simulink model "model"  (R2023b)
settings: Solver=VariableStepAuto  StartTime=0.0  StopTime=10.0  RelTol=1e-3
undefined symbols (not defined in the file): DiscIntNeverNeededParam, Newton, Raphson
libraries: simulink x43, slpidlib x11
(part 1 of 2)
settings Model: Creator=OSCAR4  LastModifiedBy=OSCAR4

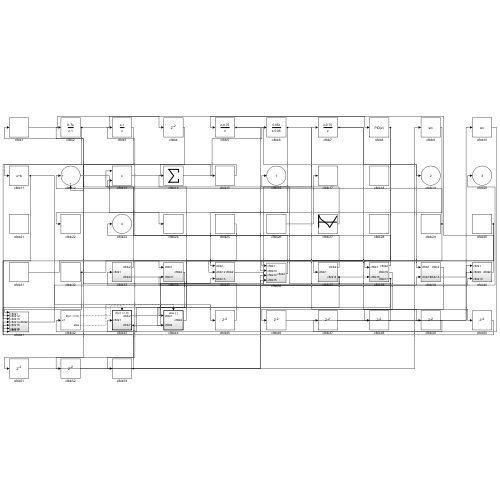
[thumbnail: Simulink's stored preview of the top-level diagram]
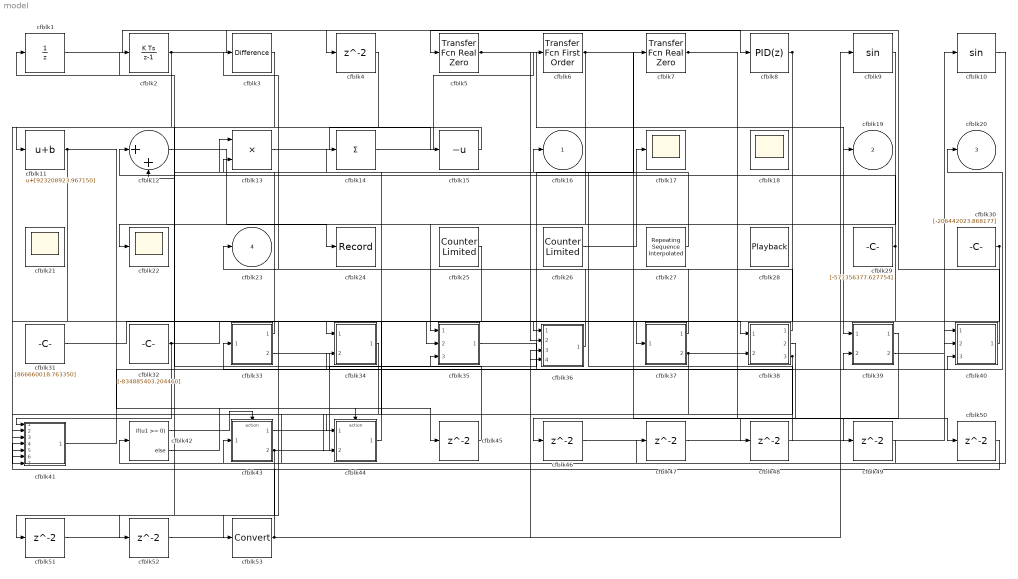
== system model ==
  cfblk1 : UnitDelay  HasFrameUpgradeWarning=on
  cfblk10 : Trigonometry
  cfblk11 : Bias  Bias=[923208923.967150]  SaturateOnIntegerOverflow=off
  cfblk12 : Sum  Inputs=|++
  cfblk13 : Product
  cfblk14 : Sum  Inputs=+
  cfblk15 : UnaryMinus
  cfblk{17..18,21..22} (4 alike) : Scope
      cfblk18 settings: Floating=on
      cfblk21 settings: Floating=on
  cfblk2 : DiscreteIntegrator  ICPrevOutput=DiscIntNeverNeededParam  ICPrevScaledInput=DiscIntNeverNeededParam
  cfblk24 : Record  FileSettingsInternal="{\"entries\":[{\"content\":{\"excelSettings\":{\"content\":{},\"type\":\"Streamout.ExcelSettings\"}},\"type\":\"Streamout.FileSettingStorage\",\"uuid\":\"\"}],\"packageUris\":[\"http:\\/\\/schema.mathworks.com\\/mf0\\/streamout_blocks\\/R2020a\"],\"version\":\"1.0\"}"  SignalsInternal="{\"entries\":[{\"content\":{\"signals\":[{\"content\":{\"blockPath\":[],\"dimensions\":[1],\"domain\":\"\",\"lineColor\":\"#ff6929\",\"plots\":[1],\"port\":1,\"sid\":[\"\"],\"signalID\":3599,\"signalName\":\"cfblk12\"},\"type\":\"RecordBlkView.Signal\",\"uuid\":\"\"}]},\"type\":\"RecordBlkView.InputSignals\",\"uuid\":\"\"}],\"packageUris\":[\"http:\\/\\/schema.mathworks.com\\/mf0\\/streamout_blocks\\/R2020a\"],\"version\":\"1.0\"}"  VisualizationBindings="{\"sparklinesplugin\":{\"info\":[{\"bindingParametersList\":[],\"subplotID\":1}]}}"
  cfblk25 : simulink/Sources/Counter Limited  uplimit=[906.000000]  tsamp=-1
  cfblk26 : simulink/Sources/Counter Limited  uplimit=[721.000000]  tsamp=-1
  cfblk27 : simulink/Sources/Repeating Sequence Interpolated  OutValues=[733850769.124770, 317296340.211416, -269417737.220056, -565735887.153496, 618114081.511135]  TimeValues=[0 0.1 0.5 0.6 1].'  LookUpMeth=Interpolation-Use End Values  tsamp=0.01  OutMin=[]  OutMax=[]  OutDataTypeStr=double  OutputDataTypeScalingMode=double  OutDataType=fixdt(0,8)  OutScaling=2^-10
  cfblk28 : Playback  NumPorts=0  PartName=b20fab14-a049-489c-adbd-99bd70615e82
  cfblk29 : Constant  Value=[-571356377.627754]  SampleTime=1
  cfblk3 : simulink/Discrete/Difference  ICPrevInput=0.0  OutMin=[]  OutMax=[]  OutDataTypeStr=Inherit: Inherit via back propagation  OutDataType=fixdt(1, 16)  OutScaling=2^-10  DoSatur=off
  cfblk30 : Constant  Value=[-206442023.868177]  SampleTime=1
  cfblk31 : Constant  Value=[866660018.763350]  SampleTime=1
  cfblk32 : Constant  Value=[-834885403.204460]  SampleTime=1
  cfblk33 : Subsystem
  cfblk34 : Subsystem
  cfblk35 : Subsystem
  cfblk36 : Subsystem
  cfblk37 : Subsystem
  cfblk38 : Subsystem
  cfblk39 : Subsystem
  cfblk{4,45..52} (9 alike) : Delay  SampleTime=1
  cfblk40 : Subsystem
  cfblk41 : Subsystem
  cfblk42 : If  IfExpression=u1 >= 0  SampleTime=1
  cfblk43 : Subsystem  TreatAsAtomicUnit=on
  cfblk44 : Subsystem  TreatAsAtomicUnit=on
  cfblk5 : simulink/Discrete/Transfer Fcn Real Zero  ZeroZ=0.75  ICPrevInput=0.0  DoSatur=off
  cfblk53 : DataTypeConversion  SaturateOnIntegerOverflow=off  RndMeth=Floor
  cfblk6 : simulink/Discrete/Transfer Fcn First Order  PoleZ=0.95  ICPrevOutput=0.0  DoSatur=off
  cfblk7 : simulink/Discrete/Transfer Fcn Real Zero  ZeroZ=0.75  ICPrevInput=0.0  DoSatur=off
  cfblk8 : slpidlib/PID Controller  Controller=PID  Form=Parallel  TimeDomain=Discrete-time  UseExternalTs=off  SampleTime=1  IntegratorMethod=Forward Euler  FilterMethod=Forward Euler  ControllerParametersSource=internal  P=1  I=1  UseKiTs=off  D=0  N=100  UseFilter=on  TunerSelectOption=Transfer Function Based (PID Tuner App)  InitialConditionSource=internal  InitialConditionForIntegrator=0  InitialConditionForFilter=0  DifferentiatorICPrevScaledInput=0  ExternalReset=none  TrackingMode=off  Kt=1  LimitOutput=off  SatLimitsSource=internal  UpperSaturationLimit=inf  LowerSaturationLimit=-inf  LinearizeAsGain=off  AntiWindupMode=none  Kb=1  LimitIntegrator=off  UpperIntegratorSaturationLimit=inf  LowerIntegratorSaturationLimit=-inf  POutMin=[]  POutMax=[]  IOutMin=[]  IOutMax=[]  DOutMin=[]  DOutMax=[]  NOutMin=[]  NOutMax=[]  SumOutMin=[]  SumOutMax=[]  SaturationOutMin=[]  SaturationOutMax=[]  PParamMin=[]  PParamMax=[]  IParamMin=[]  IParamMax=[]  DParamMin=[]  DParamMax=[]  NParamMin=[]  NParamMax=[]  KbParamMin=[]  KbParamMax=[]  KtParamMin=[]  KtParamMax=[]  KbOutMin=[]  KbOutMax=[]  KtOutMin=[]  KtOutMax=[]  IntegratorOutMin=[]  IntegratorOutMax=[]  FilterOutMin=[]  FilterOutMax=[]  SumI1OutMin=[]  SumI1OutMax=[]  SumI2OutMin=[]  SumI2OutMax=[]  SumI3OutMin=[]  SumI3OutMax=[]  SumI4OutMin=[]  SumI4OutMax=[]  SumDOutMin=[]  SumDOutMax=[]  DifferentiatorOutMin=[]  DifferentiatorOutMax=[]  FilterDiffOutCoefMin=[]  FilterDiffOutCoefMax=[]  ReciprocalOutMin=[]  ReciprocalOutMax=[]  SumDenOutMin=[]  SumDenOutMax=[]  SumNumOutMin=[]  SumNumOutMax=[]  DivideOutMin=[]  DivideOutMax=[]  UdiffTsProdOutMin=[]  UdiffTsProdOutMax=[]  NTsProdOutMin=[]  NTsProdOutMax=[]  UintegralTsProdOutMin=[]  UintegralTsProdOutMax=[]  UngainTsProdOutMin=[]  UngainTsProdOutMax=[]  ClampingZeroOutDataTypeStr=Inherit: Inherit via back propagation  ClampingZeroOutMin=[]  ClampingZeroOutMax=[]  FilterDenConstantOutDataTypeStr=Inherit: Inherit via back propagation  FilterDenConstantOutMin=[]  FilterDenConstantOutMax=[]  PCopyOutDataTypeStr=Inherit: Inherit via back propagation  PCopyOutMin=[]  PCopyOutMax=[]  NCopyOutDataTypeStr=Inherit: Inherit via back propagation  NCopyOutMin=[]  NCopyOutMax=[]  IntegratorContinuousStateAttributes=''  IntegratorStateMustResolveToSignalObject=off  IntegratorRTWStateStorageClass=Auto  FilterContinuousStateAttributes=''  FilterStateMustResolveToSignalObject=off  FilterRTWStateStorageClass=Auto  ParallelPVariant=InternalParameters  IdealPVariant=Disabled  IVariant=InternalParameters  DVariant=InternalParameters  IntegratorVariant=Discrete  SatVariant=Disabled  AWVariant=Passthrough  PCopyVariant=Disabled  TRVariant=Disabled  FdbkBlocksVariant=Forward  IdealPFdbkVariant=Disabled  SatFdbkVariant=Disabled  DerivativeFilterVariant=ForwardEulerFilter  NVariant=InternalParameters  NCopyVariant=Disabled  FilterICVariant=InternalICsFilter  IntegratorICVariant=InternalICs  ExternalResetVariant=Disabled  TRSumVariant=Passthrough  SumFdbkVariant=Disabled  SumVariant=Sum_PID  TsampFilterVariant=InternalTs  TsampNgainVariant=Passthrough  TsampIntegralVariant=Disabled_SignalSpec  ExternalSaturationOutDataTypeStr=Inherit: Same as second input
      settings: LibrarySourceBlock=simulink/Discrete/Discrete PID Controller
  cfblk9 : Trigonometry
  cfblk16 : Outport
  cfblk19 : Outport  Port=2
  cfblk20 : Outport  Port=3
  cfblk23 : Outport  Port=4
  wires:
  cfblk9/1 -> cfblk35/1(cfblk1)
  cfblk33/1(cfblk2) -> cfblk1/1
  cfblk27/1 -> cfblk16/1
  cfblk40/1(cfblk2) -> cfblk5/1
  cfblk6/1 -> cfblk49/1, cfblk52/1
  cfblk26/1 -> cfblk17/1
  cfblk2/1 -> cfblk8/1, cfblk41/3(cfblk13)
  cfblk8/1 -> cfblk35/2(cfblk12), cfblk36/1(cfblk1)
  cfblk12/1 -> cfblk24/1
  cfblk32/1 -> cfblk41/1(cfblk1), cfblk36/2(cfblk13)
  cfblk31/1 -> cfblk34/1(cfblk1)
  cfblk29/1 -> cfblk12/1, cfblk41/6(cfblk16)
  cfblk5/1 -> cfblk39/1(cfblk1), cfblk38/1(cfblk1)
  cfblk34/1(cfblk2) -> cfblk42/1
  cfblk25/1 -> cfblk53/1
  cfblk7/1 -> cfblk19/1, cfblk50/1
  cfblk35/1(cfblk2) -> cfblk20/1
  cfblk1/1 -> cfblk4/1
  cfblk11/1 -> cfblk41/7(cfblk17), cfblk45/1
  cfblk14/1 -> cfblk6/1
  cfblk43/1(cfblk2) -> cfblk35/3(cfblk13)
  cfblk4/1 -> cfblk12/2
  cfblk15/1 -> cfblk11/1
  cfblk3/1 -> cfblk22/1
  cfblk13/1 -> cfblk15/1
  cfblk39/2(cfblk16) -> cfblk10/1
  cfblk43/2(cfblk7) -> cfblk7/1, cfblk51/1
  cfblk33/2(cfblk9) -> cfblk39/2(cfblk15)
  cfblk41/1(cfblk2) -> cfblk40/3(cfblk10)
  cfblk30/1 -> cfblk44/1(cfblk1), cfblk37/1(cfblk1)
  cfblk38/1(cfblk2) -> cfblk23/1
  cfblk37/1(cfblk2) -> cfblk3/1
  cfblk38/3(cfblk17) -> cfblk33/1(cfblk1), cfblk44/2(cfblk9)
  cfblk37/2(cfblk14) -> cfblk34/2(cfblk11), cfblk38/2(cfblk15), cfblk41/2(cfblk12)
  cfblk44/1(cfblk2) -> cfblk14/1
  cfblk36/1(cfblk2) -> cfblk13/2
  cfblk42/1 -> cfblk43/Action
  cfblk42/2 -> cfblk44/Action
  cfblk45/1 -> cfblk2/1
  cfblk39/1(cfblk2) -> cfblk46/1
  cfblk46/1 -> cfblk40/1(cfblk1)
  cfblk10/1 -> cfblk47/1
  cfblk47/1 -> cfblk40/2(cfblk9)
  cfblk38/2(cfblk16) -> cfblk48/1
  cfblk48/1 -> cfblk13/1
  cfblk49/1 -> cfblk43/1(cfblk1)
  cfblk50/1 -> cfblk41/4(cfblk14)
  cfblk51/1 -> cfblk36/3(cfblk14)
  cfblk52/1 -> cfblk36/4(cfblk15)
  cfblk53/1 -> cfblk41/5(cfblk15), cfblk9/1

== system model/cfblk33 ==
  cfblk1 : Inport
  cfblk{10..15} (6 alike) : Delay  SampleTime=1
  cfblk3 : Bias  Bias=[280555499.209251]  SaturateOnIntegerOverflow=off
  cfblk4 : simulink/Math Operations/Slider Gain  gain=1  low=0  high=2
  cfblk5 : Subsystem
  cfblk6 : Subsystem
  cfblk7 : Subsystem
  cfblk8 : Subsystem
  cfblk2 : Outport
  cfblk9 : Outport  Port=2
  wires:
  cfblk4/1 -> cfblk9/1
  cfblk1/1 -> cfblk7/1(cfblk1)
  cfblk7/1(cfblk2) -> cfblk6/1(cfblk1)
  cfblk6/1(cfblk2) -> cfblk3/1, cfblk8/3(cfblk13), cfblk5/2(cfblk8), cfblk2/1
  cfblk8/1(cfblk2) -> cfblk5/1(cfblk1)
  cfblk5/3(cfblk10) -> cfblk12/1, cfblk13/1
  cfblk8/2(cfblk15) -> cfblk14/1, cfblk15/1
  cfblk3/1 -> cfblk4/1
  cfblk5/1(cfblk2) -> cfblk10/1
  cfblk10/1 -> cfblk8/1(cfblk1)
  cfblk5/2(cfblk9) -> cfblk11/1
  cfblk11/1 -> cfblk8/2(cfblk12)
  cfblk12/1 -> cfblk7/2(cfblk14)
  cfblk13/1 -> cfblk8/4(cfblk14)
  cfblk14/1 -> cfblk7/3(cfblk15)
  cfblk15/1 -> cfblk7/4(cfblk16)

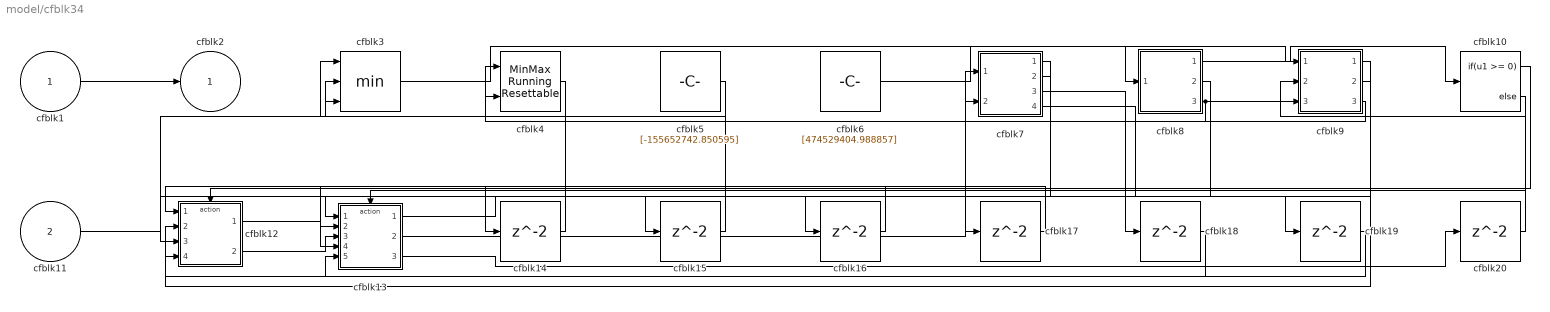
== system model/cfblk34 ==
  cfblk1 : Inport
  cfblk11 : Inport  Port=2
  cfblk10 : If  IfExpression=u1 >= 0  SampleTime=1
  cfblk12 : Subsystem  TreatAsAtomicUnit=on
  cfblk13 : Subsystem  TreatAsAtomicUnit=on
  cfblk{14..20} (7 alike) : Delay  SampleTime=1
  cfblk3 : MinMax  Inputs=3
  cfblk4 : simulink/Math Operations/MinMax Running Resettable  Function=min  vinit=0.0
  cfblk5 : Constant  Value=[-155652742.850595]  SampleTime=1
  cfblk6 : Constant  Value=[474529404.988857]  SampleTime=1
  cfblk7 : Subsystem
  cfblk8 : Subsystem
  cfblk9 : Subsystem
  cfblk2 : Outport
  wires:
  cfblk4/1 -> cfblk13/1(cfblk1)
  cfblk1/1 -> cfblk2/1
  cfblk12/2(cfblk12) -> cfblk13/3(cfblk11)
  cfblk5/1 -> cfblk3/2
  cfblk9/1(cfblk2) -> cfblk12/2(cfblk9)
  cfblk8/1(cfblk2) -> cfblk10/1
  cfblk6/1 -> cfblk8/1(cfblk1)
  cfblk8/2(cfblk9) -> cfblk12/3(cfblk10)
  cfblk13/2(cfblk14) -> cfblk7/1(cfblk1)
  cfblk9/2(cfblk8) -> cfblk13/4(cfblk12)
  cfblk3/1 -> cfblk9/1(cfblk1)
  cfblk11/1 -> cfblk4/1
  cfblk8/3(cfblk10) -> cfblk9/3(cfblk7), cfblk7/2(cfblk7)
  cfblk9/3(cfblk9) -> cfblk4/2
  cfblk10/1 -> cfblk12/Action
  cfblk10/2 -> cfblk13/Action
  cfblk12/1(cfblk2) -> cfblk14/1
  cfblk14/1 -> cfblk3/1
  cfblk13/1(cfblk2) -> cfblk15/1
  cfblk15/1 -> cfblk3/3
  cfblk7/1(cfblk2) -> cfblk16/1
  cfblk16/1 -> cfblk12/1(cfblk1)
  cfblk7/2(cfblk8) -> cfblk17/1
  cfblk17/1 -> cfblk13/2(cfblk10)
  cfblk7/3(cfblk9) -> cfblk18/1
  cfblk18/1 -> cfblk12/4(cfblk11)
  cfblk7/4(cfblk10) -> cfblk19/1
  cfblk19/1 -> cfblk13/5(cfblk13)
  cfblk13/3(cfblk15) -> cfblk20/1
  cfblk20/1 -> cfblk9/2(cfblk6)

== system model/cfblk35 ==
  cfblk1 : Inport
  cfblk12 : Inport  Port=2
  cfblk13 : Inport  Port=3
  cfblk10 : Subsystem
  cfblk11 : Subsystem
  cfblk{3,14..16} (4 alike) : Delay  SampleTime=1
  cfblk4 : UnitDelay  HasFrameUpgradeWarning=on
  cfblk5 : UnitDelay  HasFrameUpgradeWarning=on
  cfblk6 : Abs  SaturateOnIntegerOverflow=off
  cfblk7 : Sqrt  Operator=rSqrt  AlgorithmType=Newton-Raphson
  cfblk8 : ComplexToMagnitudeAngle
  cfblk9 : Constant  Value=[-846214747.053952]  SampleTime=1
  cfblk2 : Outport
  wires:
  cfblk3/1 -> cfblk5/1
  cfblk9/1 -> cfblk10/1(cfblk1)
  cfblk5/1 -> cfblk7/1
  cfblk11/1(cfblk2) -> cfblk2/1, cfblk10/7(cfblk15)
  cfblk12/1 -> cfblk11/1(cfblk1)
  cfblk7/1 -> cfblk10/4(cfblk12), cfblk16/1
  cfblk6/1 -> cfblk11/2(cfblk15), cfblk10/6(cfblk14)
  cfblk10/1(cfblk2) -> cfblk8/1
  cfblk8/1 -> cfblk4/1
  cfblk13/1 -> cfblk11/3(cfblk16), cfblk10/5(cfblk13)
  cfblk1/1 -> cfblk6/1
  cfblk4/1 -> cfblk14/1
  cfblk14/1 -> cfblk10/2(cfblk10)
  cfblk8/2 -> cfblk15/1
  cfblk15/1 -> cfblk10/3(cfblk11)
  cfblk16/1 -> cfblk3/1

== system model/cfblk36 ==
  cfblk1 : Inport
  cfblk13 : Inport  Port=2
  cfblk14 : Inport  Port=3
  cfblk15 : Inport  Port=4
  cfblk10 : Subsystem
  cfblk11 : Subsystem
  cfblk12 : Subsystem
  cfblk16 : Delay  SampleTime=1
  cfblk3 : Delay  ShowEnablePort=on  SampleTime=1
      settings: InputPortMap=u0,e6
  cfblk4 : DotProduct  OutDataTypeStr=Inherit: Inherit via internal rule
  cfblk5 : Sum  Inputs=+-
  cfblk6 : Bias  Bias=[-194164036.502314]  SaturateOnIntegerOverflow=off
  cfblk7 : simulink/Math Operations/MinMax Running Resettable  Function=min  vinit=0.0
  cfblk8 : Gain  Gain=[756991828.440639]
  cfblk9 : Constant  Value=[963201861.308035]  SampleTime=1
  cfblk2 : Outport
  wires:
  cfblk10/1(cfblk2) -> cfblk7/1
  cfblk13/1 -> cfblk3/1
  cfblk11/1(cfblk2) -> cfblk6/1
  cfblk7/1 -> cfblk12/1(cfblk1)
  cfblk6/1 -> cfblk2/1
  cfblk3/1 -> cfblk11/1(cfblk1)
  cfblk10/2(cfblk6) -> cfblk5/1
  cfblk11/2(cfblk13) -> cfblk7/2
  cfblk8/1 -> cfblk4/1
  cfblk14/1 -> cfblk4/2
  cfblk1/1 -> cfblk10/1(cfblk1)
  cfblk9/1 -> cfblk11/2(cfblk12)
  cfblk15/1 -> cfblk12/2(cfblk5)
  cfblk10/3(cfblk7) -> cfblk3/2
  cfblk4/1 -> cfblk5/2
  cfblk10/4(cfblk8) -> cfblk12/3(cfblk6)
  cfblk10/5(cfblk9) -> cfblk12/5(cfblk8)
  cfblk12/1(cfblk2) -> cfblk8/1
  cfblk5/1 -> cfblk16/1
  cfblk16/1 -> cfblk12/4(cfblk7)

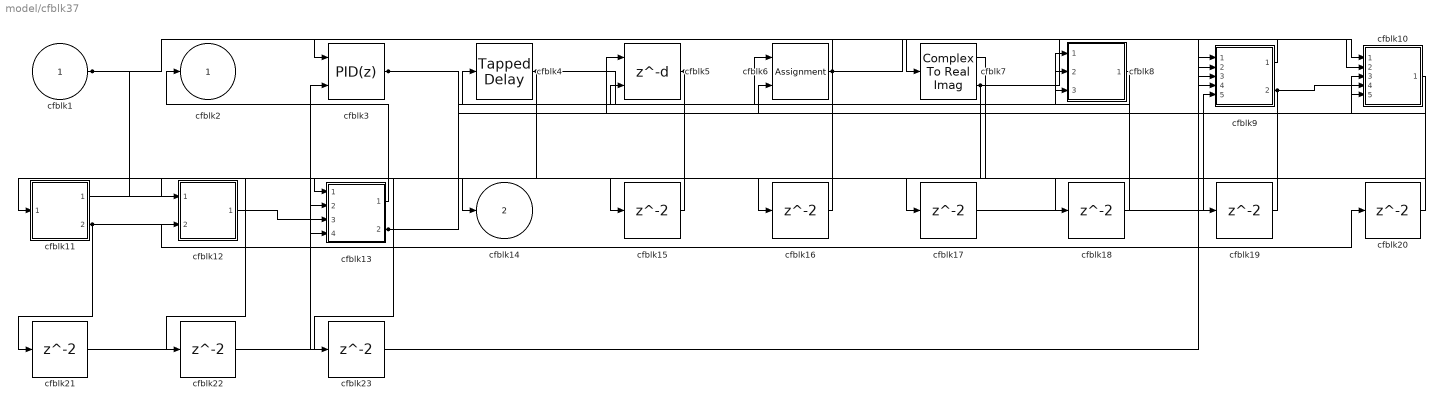
== system model/cfblk37 ==
  cfblk1 : Inport
  cfblk10 : Subsystem
  cfblk11 : Subsystem
  cfblk12 : Subsystem
  cfblk13 : Subsystem
  cfblk{15..23} (9 alike) : Delay  SampleTime=1
  cfblk3 : slpidlib/PID Controller (2DOF)  Controller=PID  Form=Parallel  TimeDomain=Discrete-time  UseExternalTs=off  SampleTime=1  IntegratorMethod=Forward Euler  FilterMethod=Forward Euler  ControllerParametersSource=internal  P=1  I=1  UseKiTs=off  D=0  N=100  UseFilter=on  b=1  c=1  TunerSelectOption=Transfer Function Based (PID Tuner App)  InitialConditionSource=internal  InitialConditionForIntegrator=0  InitialConditionForFilter=0  DifferentiatorICPrevScaledInput=0  ExternalReset=none  TrackingMode=off  Kt=1  LimitOutput=off  SatLimitsSource=internal  UpperSaturationLimit=inf  LowerSaturationLimit=-inf  LinearizeAsGain=off  AntiWindupMode=none  Kb=1  LimitIntegrator=off  UpperIntegratorSaturationLimit=inf  LowerIntegratorSaturationLimit=-inf  POutMin=[]  POutMax=[]  IOutMin=[]  IOutMax=[]  DOutMin=[]  DOutMax=[]  NOutMin=[]  NOutMax=[]  bOutMin=[]  bOutMax=[]  cOutMin=[]  cOutMax=[]  SumOutMin=[]  SumOutMax=[]  SaturationOutMin=[]  SaturationOutMax=[]  PParamMin=[]  PParamMax=[]  IParamMin=[]  IParamMax=[]  DParamMin=[]  DParamMax=[]  NParamMin=[]  NParamMax=[]  bParamMin=[]  bParamMax=[]  cParamMin=[]  cParamMax=[]  KbParamMin=[]  KbParamMax=[]  KtParamMin=[]  KtParamMax=[]  KbOutMin=[]  KbOutMax=[]  KtOutMin=[]  KtOutMax=[]  IntegratorOutMin=[]  IntegratorOutMax=[]  FilterOutMin=[]  FilterOutMax=[]  SumI1OutMin=[]  SumI1OutMax=[]  SumI2OutMin=[]  SumI2OutMax=[]  SumI3OutMin=[]  SumI3OutMax=[]  SumI4OutMin=[]  SumI4OutMax=[]  SumDOutMin=[]  SumDOutMax=[]  Sum1OutMin=[]  Sum1OutMax=[]  Sum2OutMin=[]  Sum2OutMax=[]  Sum3OutMin=[]  Sum3OutMax=[]  DifferentiatorOutMin=[]  DifferentiatorOutMax=[]  FilterDiffOutCoefMin=[]  FilterDiffOutCoefMax=[]  ReciprocalOutMin=[]  ReciprocalOutMax=[]  SumDenOutMin=[]  SumDenOutMax=[]  SumNumOutMin=[]  SumNumOutMax=[]  DivideOutMin=[]  DivideOutMax=[]  UdiffTsProdOutMin=[]  UdiffTsProdOutMax=[]  NTsProdOutMin=[]  NTsProdOutMax=[]  UintegralTsProdOutMin=[]  UintegralTsProdOutMax=[]  UngainTsProdOutMin=[]  UngainTsProdOutMax=[]  ClampingZeroOutDataTypeStr=Inherit: Inherit via back propagation  ClampingZeroOutMin=[]  ClampingZeroOutMax=[]  FilterDenConstantOutDataTypeStr=Inherit: Inherit via back propagation  FilterDenConstantOutMin=[]  FilterDenConstantOutMax=[]  PCopyOutDataTypeStr=Inherit: Inherit via back propagation  PCopyOutMin=[]  PCopyOutMax=[]  NCopyOutDataTypeStr=Inherit: Inherit via back propagation  NCopyOutMin=[]  NCopyOutMax=[]  IntegratorContinuousStateAttributes=''  IntegratorStateMustResolveToSignalObject=off  IntegratorRTWStateStorageClass=Auto  FilterContinuousStateAttributes=''  FilterStateMustResolveToSignalObject=off  FilterRTWStateStorageClass=Auto  ParallelPVariant=InternalParameters  IdealPVariant=Disabled  IVariant=InternalParameters  DVariant=InternalParameters  bVariant=InternalParameters  cVariant=InternalParameters  IntegratorVariant=Discrete  SatVariant=Disabled  AWVariant=Passthrough  PCopyVariant=Disabled  TRVariant=Disabled  FdbkBlocksVariant=Forward  IdealPFdbkVariant=Disabled  SatFdbkVariant=Disabled  DerivativeFilterVariant=ForwardEulerFilter  NVariant=InternalParameters  NCopyVariant=Disabled  FilterICVariant=InternalICsFilter  IntegratorICVariant=InternalICs  ExternalResetVariant=Disabled  TRSumVariant=Passthrough  SumFdbkVariant=Disabled  SumVariant=Sum_PID  TsampFilterVariant=InternalTs  TsampNgainVariant=Passthrough  TsampIntegralVariant=Disabled_SignalSpec  ExternalSaturationOutDataTypeStr=Inherit: Same as second input
      settings: LibrarySourceBlock=simulink/Discrete/Discrete PID Controller (2DOF)
  cfblk4 : simulink/Discrete/Tapped Delay  vinit=0.0  samptime=-1  NumDelays=1  DelayOrder=Oldest  includeCurrent=off
  cfblk5 : Delay  DelayLengthSource=Input port  SampleTime=1
      settings: InputPortMap=u0,p1
  cfblk6 : Assignment  DiagnosticForDimensions=Warning  IndexOptions=Index vector (dialog)  Indices=1  OutputSizes=1
  cfblk7 : ComplexToRealImag
  cfblk8 : Subsystem
  cfblk9 : Subsystem
  cfblk2 : Outport
  cfblk14 : Outport  Port=2
  wires:
  cfblk7/1 -> cfblk14/1
  cfblk1/1 -> cfblk12/1(cfblk1), cfblk9/2(cfblk8)
  cfblk5/1 -> cfblk4/1, cfblk13/4(cfblk13), cfblk22/1
  cfblk9/1(cfblk2) -> cfblk7/1
  cfblk6/1 -> cfblk3/1, cfblk10/2(cfblk13), cfblk23/1
  cfblk7/2 -> cfblk10/1(cfblk1), cfblk17/1
  cfblk11/2(cfblk17) -> cfblk12/2(cfblk16), cfblk20/1, cfblk21/1
  cfblk3/1 -> cfblk5/2, cfblk18/1
  cfblk4/1 -> cfblk11/1(cfblk1), cfblk8/3(cfblk10)
  cfblk9/2(cfblk12) -> cfblk6/2, cfblk10/4(cfblk15)
  cfblk13/1(cfblk2) -> cfblk2/1
  cfblk12/1(cfblk2) -> cfblk13/3(cfblk12)
  cfblk13/2(cfblk14) -> cfblk8/1(cfblk1), cfblk10/3(cfblk14), cfblk10/5(cfblk16), cfblk8/2(cfblk9)
  cfblk8/1(cfblk2) -> cfblk15/1
  cfblk15/1 -> cfblk13/2(cfblk11)
  cfblk10/1(cfblk2) -> cfblk16/1
  cfblk16/1 -> cfblk13/1(cfblk1)
  cfblk17/1 -> cfblk9/5(cfblk11)
  cfblk18/1 -> cfblk6/1
  cfblk11/1(cfblk2) -> cfblk19/1
  cfblk19/1 -> cfblk9/1(cfblk1)
  cfblk20/1 -> cfblk5/1
  cfblk21/1 -> cfblk3/2
  cfblk22/1 -> cfblk9/3(cfblk9)
  cfblk23/1 -> cfblk9/4(cfblk10)

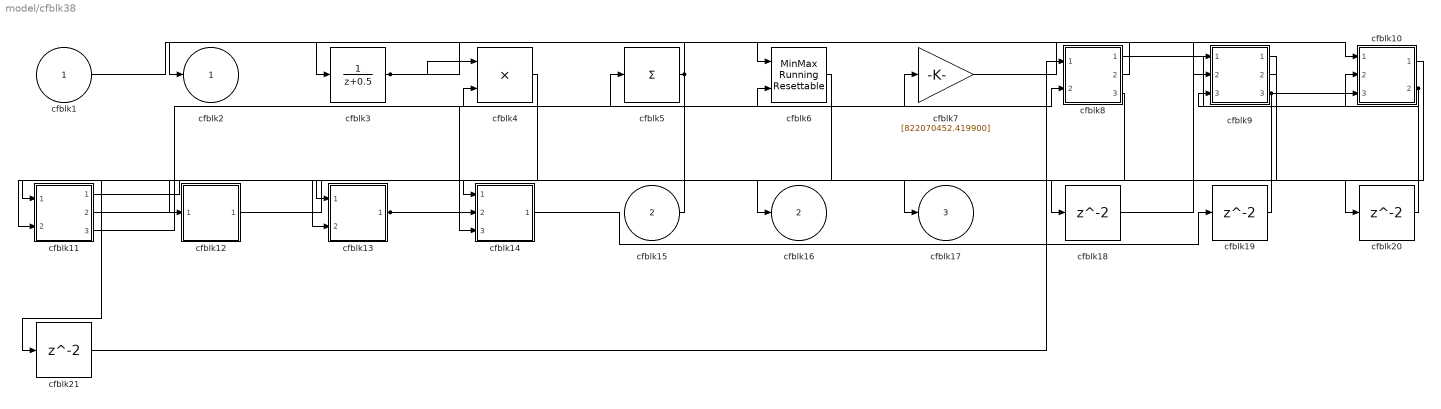
== system model/cfblk38 ==
  cfblk1 : Inport
  cfblk15 : Inport  Port=2
  cfblk10 : Subsystem
  cfblk11 : Subsystem
  cfblk12 : Subsystem
  cfblk13 : Subsystem
  cfblk14 : Subsystem
  cfblk{18..21} (4 alike) : Delay  SampleTime=1
  cfblk3 : DiscreteTransferFcn  SampleTime=1
  cfblk4 : Product  Inputs=**
  cfblk5 : Sum  Inputs=+
  cfblk6 : simulink/Math Operations/MinMax Running Resettable  Function=min  vinit=0.0
  cfblk7 : Gain  Gain=[822070452.419900]
  cfblk8 : Subsystem
  cfblk9 : Subsystem
  cfblk2 : Outport
  cfblk16 : Outport  Port=2
  cfblk17 : Outport  Port=3
  wires:
  cfblk6/1 -> cfblk16/1
  cfblk12/1(cfblk2) -> cfblk14/1(cfblk1)
  cfblk7/1 -> cfblk10/1(cfblk1)
  cfblk5/1 -> cfblk2/1, cfblk4/2
  cfblk8/1(cfblk2) -> cfblk10/2(cfblk12)
  cfblk8/2(cfblk10) -> cfblk3/1
  cfblk1/1 -> cfblk9/2(cfblk7)
  cfblk13/1(cfblk2) -> cfblk6/2, cfblk20/1
  cfblk15/1 -> cfblk5/1
  cfblk10/1(cfblk2) -> cfblk14/2(cfblk14)
  cfblk11/2(cfblk8) -> cfblk8/2(cfblk9)
  cfblk11/3(cfblk9) -> cfblk7/1
  cfblk9/1(cfblk2) -> cfblk11/2(cfblk7)
  cfblk9/2(cfblk9) -> cfblk12/1(cfblk1)
  cfblk8/3(cfblk11) -> cfblk14/3(cfblk15)
  cfblk9/3(cfblk10) -> cfblk10/3(cfblk13), cfblk17/1
  cfblk10/2(cfblk14) -> cfblk13/1(cfblk1), cfblk13/2(cfblk17)
  cfblk3/1 -> cfblk4/1, cfblk6/1
  cfblk11/1(cfblk2) -> cfblk18/1
  cfblk18/1 -> cfblk9/1(cfblk1)
  cfblk14/1(cfblk2) -> cfblk19/1
  cfblk19/1 -> cfblk11/1(cfblk1)
  cfblk20/1 -> cfblk9/3(cfblk8)
  cfblk4/1 -> cfblk21/1
  cfblk21/1 -> cfblk8/1(cfblk1)

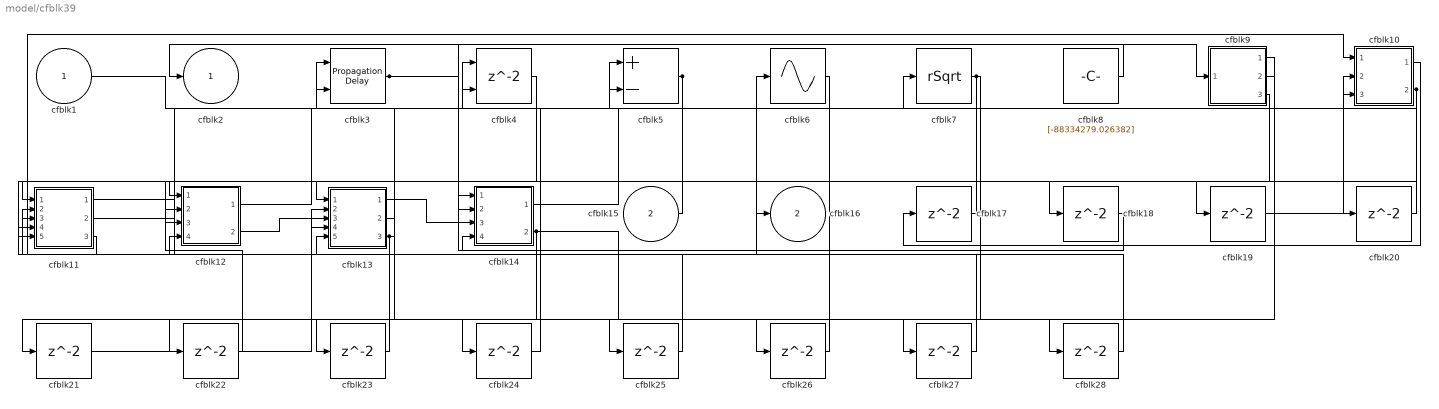
== system model/cfblk39 ==
  cfblk1 : Inport
  cfblk15 : Inport  Port=2
  cfblk10 : Subsystem
  cfblk11 : Subsystem
  cfblk12 : Subsystem
  cfblk13 : Subsystem
  cfblk14 : Subsystem
  cfblk{17..28} (12 alike) : Delay  SampleTime=1
  cfblk3 : PropagationDelay  SampleTime=1
  cfblk4 : Delay  ShowEnablePort=on  SampleTime=1
      settings: InputPortMap=u0,e6
  cfblk5 : Sum  Inputs=+-
  cfblk6 : Sin  TimeSource=Use external signal  SampleTime=0
  cfblk7 : Sqrt  Operator=rSqrt  AlgorithmType=Newton-Raphson
  cfblk8 : Constant  Value=[-88334279.026382]  SampleTime=1
  cfblk9 : Subsystem
  cfblk2 : Outport
  cfblk16 : Outport  Port=2
  wires:
  cfblk8/1 -> cfblk2/1
  cfblk15/1 -> cfblk5/1
  cfblk11/1(cfblk2) -> cfblk6/1
  cfblk4/1 -> cfblk13/1(cfblk1)
  cfblk7/1 -> cfblk26/1, cfblk27/1
  cfblk11/2(cfblk13) -> cfblk7/1
  cfblk11/3(cfblk14) -> cfblk10/1(cfblk1)
  cfblk12/1(cfblk2) -> cfblk4/1
  cfblk13/1(cfblk2) -> cfblk14/3(cfblk9)
  cfblk14/1(cfblk2) -> cfblk10/2(cfblk11)
  cfblk14/2(cfblk11) -> cfblk11/3(cfblk10), cfblk24/1, cfblk28/1
  cfblk1/1 -> cfblk5/2
  cfblk10/2(cfblk13) -> cfblk3/1, cfblk18/1
  cfblk13/2(cfblk16) -> cfblk11/1(cfblk1)
  cfblk3/1 -> cfblk9/1(cfblk1), cfblk16/1, cfblk19/1, cfblk20/1
  cfblk5/1 -> cfblk12/1(cfblk1), cfblk11/5(cfblk12)
  cfblk12/2(cfblk13) -> cfblk13/3(cfblk13)
  cfblk13/3(cfblk17) -> cfblk11/2(cfblk9), cfblk3/2
  cfblk10/1(cfblk2) -> cfblk17/1
  cfblk17/1 -> cfblk14/2(cfblk8)
  cfblk18/1 -> cfblk14/4(cfblk10)
  cfblk19/1 -> cfblk10/3(cfblk12)
  cfblk20/1 -> cfblk12/3(cfblk11)
  cfblk9/1(cfblk2) -> cfblk21/1
  cfblk21/1 -> cfblk13/4(cfblk14)
  cfblk9/2(cfblk15) -> cfblk22/1
  cfblk22/1 -> cfblk12/2(cfblk10)
  cfblk9/3(cfblk16) -> cfblk23/1
  cfblk23/1 -> cfblk13/5(cfblk15)
  cfblk24/1 -> cfblk4/2
  cfblk6/1 -> cfblk25/1
  cfblk25/1 -> cfblk13/2(cfblk12)
  cfblk26/1 -> cfblk14/1(cfblk1)
  cfblk27/1 -> cfblk11/4(cfblk11)
  cfblk28/1 -> cfblk12/4(cfblk12)

== system model/cfblk40 ==
  cfblk1 : Inport
  cfblk9 : Inport  Port=2
  cfblk10 : Inport  Port=3
  cfblk11 : Subsystem  TreatAsAtomicUnit=on
  cfblk12 : Subsystem  TreatAsAtomicUnit=on
  cfblk{13..16} (4 alike) : Delay  SampleTime=1
  cfblk3 : Sqrt
  cfblk4 : UnaryMinus
  cfblk5 : Sum  Inputs=+-
  cfblk6 : Subsystem
  cfblk7 : Subsystem
  cfblk8 : If  IfExpression=u1 >= 0  SampleTime=1
  cfblk2 : Outport
  wires:
  cfblk9/1 -> cfblk8/1
  cfblk11/1(cfblk2) -> cfblk3/1
  cfblk3/1 -> cfblk6/1(cfblk1)
  cfblk7/1(cfblk2) -> cfblk4/1
  cfblk1/1 -> cfblk11/1(cfblk1)
  cfblk10/1 -> cfblk6/2(cfblk5)
  cfblk11/2(cfblk11) -> cfblk5/1
  cfblk5/1 -> cfblk2/1
  cfblk6/1(cfblk2) -> cfblk5/2
  cfblk6/3(cfblk8) -> cfblk7/2(cfblk12), cfblk16/1
  cfblk12/1(cfblk2) -> cfblk7/3(cfblk13)
  cfblk8/1 -> cfblk11/Action
  cfblk8/2 -> cfblk12/Action
  cfblk6/2(cfblk7) -> cfblk13/1
  cfblk13/1 -> cfblk12/1(cfblk1)
  cfblk4/1 -> cfblk14/1
  cfblk14/1 -> cfblk7/1(cfblk1)
  cfblk7/2(cfblk14) -> cfblk15/1
  cfblk15/1 -> cfblk6/3(cfblk6)
  cfblk16/1 -> cfblk12/2(cfblk5)

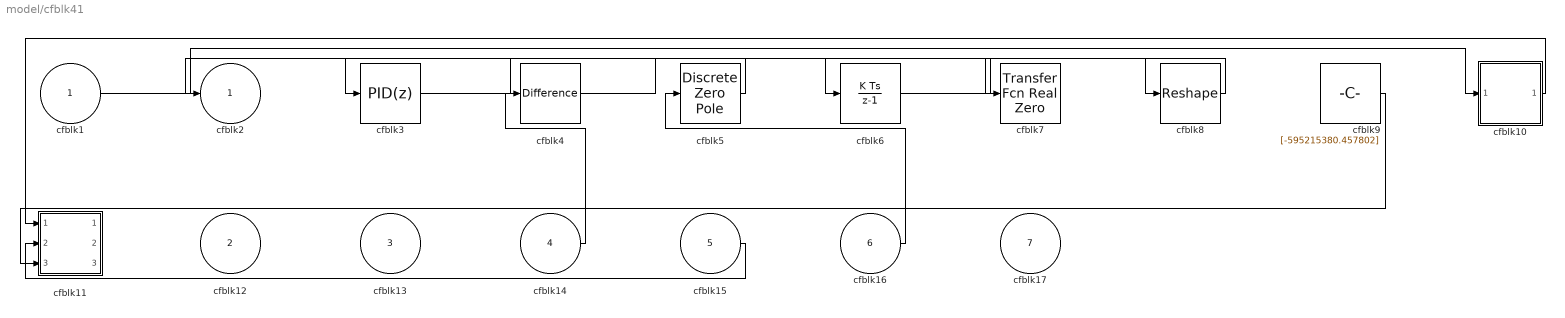
== system model/cfblk41 ==
  cfblk1 : Inport
  cfblk12 : Inport  Port=2
  cfblk13 : Inport  Port=3
  cfblk14 : Inport  Port=4
  cfblk15 : Inport  Port=5
  cfblk16 : Inport  Port=6
  cfblk17 : Inport  Port=7
  cfblk10 : Subsystem
  cfblk11 : Subsystem
  cfblk3 : slpidlib/PID Controller  Controller=PID  Form=Parallel  TimeDomain=Discrete-time  UseExternalTs=off  SampleTime=1  IntegratorMethod=Forward Euler  FilterMethod=Forward Euler  ControllerParametersSource=internal  P=1  I=1  UseKiTs=off  D=0  N=100  UseFilter=on  TunerSelectOption=Transfer Function Based (PID Tuner App)  InitialConditionSource=internal  InitialConditionForIntegrator=0  InitialConditionForFilter=0  DifferentiatorICPrevScaledInput=0  ExternalReset=none  TrackingMode=off  Kt=1  LimitOutput=off  SatLimitsSource=internal  UpperSaturationLimit=inf  LowerSaturationLimit=-inf  LinearizeAsGain=off  AntiWindupMode=none  Kb=1  LimitIntegrator=off  UpperIntegratorSaturationLimit=inf  LowerIntegratorSaturationLimit=-inf  POutMin=[]  POutMax=[]  IOutMin=[]  IOutMax=[]  DOutMin=[]  DOutMax=[]  NOutMin=[]  NOutMax=[]  SumOutMin=[]  SumOutMax=[]  SaturationOutMin=[]  SaturationOutMax=[]  PParamMin=[]  PParamMax=[]  IParamMin=[]  IParamMax=[]  DParamMin=[]  DParamMax=[]  NParamMin=[]  NParamMax=[]  KbParamMin=[]  KbParamMax=[]  KtParamMin=[]  KtParamMax=[]  KbOutMin=[]  KbOutMax=[]  KtOutMin=[]  KtOutMax=[]  IntegratorOutMin=[]  IntegratorOutMax=[]  FilterOutMin=[]  FilterOutMax=[]  SumI1OutMin=[]  SumI1OutMax=[]  SumI2OutMin=[]  SumI2OutMax=[]  SumI3OutMin=[]  SumI3OutMax=[]  SumI4OutMin=[]  SumI4OutMax=[]  SumDOutMin=[]  SumDOutMax=[]  DifferentiatorOutMin=[]  DifferentiatorOutMax=[]  FilterDiffOutCoefMin=[]  FilterDiffOutCoefMax=[]  ReciprocalOutMin=[]  ReciprocalOutMax=[]  SumDenOutMin=[]  SumDenOutMax=[]  SumNumOutMin=[]  SumNumOutMax=[]  DivideOutMin=[]  DivideOutMax=[]  UdiffTsProdOutMin=[]  UdiffTsProdOutMax=[]  NTsProdOutMin=[]  NTsProdOutMax=[]  UintegralTsProdOutMin=[]  UintegralTsProdOutMax=[]  UngainTsProdOutMin=[]  UngainTsProdOutMax=[]  ClampingZeroOutDataTypeStr=Inherit: Inherit via back propagation  ClampingZeroOutMin=[]  ClampingZeroOutMax=[]  FilterDenConstantOutDataTypeStr=Inherit: Inherit via back propagation  FilterDenConstantOutMin=[]  FilterDenConstantOutMax=[]  PCopyOutDataTypeStr=Inherit: Inherit via back propagation  PCopyOutMin=[]  PCopyOutMax=[]  NCopyOutDataTypeStr=Inherit: Inherit via back propagation  NCopyOutMin=[]  NCopyOutMax=[]  IntegratorContinuousStateAttributes=''  IntegratorStateMustResolveToSignalObject=off  IntegratorRTWStateStorageClass=Auto  FilterContinuousStateAttributes=''  FilterStateMustResolveToSignalObject=off  FilterRTWStateStorageClass=Auto  ParallelPVariant=InternalParameters  IdealPVariant=Disabled  IVariant=InternalParameters  DVariant=InternalParameters  IntegratorVariant=Discrete  SatVariant=Disabled  AWVariant=Passthrough  PCopyVariant=Disabled  TRVariant=Disabled  FdbkBlocksVariant=Forward  IdealPFdbkVariant=Disabled  SatFdbkVariant=Disabled  DerivativeFilterVariant=ForwardEulerFilter  NVariant=InternalParameters  NCopyVariant=Disabled  FilterICVariant=InternalICsFilter  IntegratorICVariant=InternalICs  ExternalResetVariant=Disabled  TRSumVariant=Passthrough  SumFdbkVariant=Disabled  SumVariant=Sum_PID  TsampFilterVariant=InternalTs  TsampNgainVariant=Passthrough  TsampIntegralVariant=Disabled_SignalSpec  ExternalSaturationOutDataTypeStr=Inherit: Same as second input
      settings: LibrarySourceBlock=simulink/Discrete/Discrete PID Controller
  cfblk4 : simulink/Discrete/Difference  ICPrevInput=0.0  OutMin=[]  OutMax=[]  OutDataTypeStr=Inherit: Inherit via back propagation  OutDataType=fixdt(1, 16)  OutScaling=2^-10  DoSatur=off
  cfblk5 : DiscreteZeroPole  Poles=[0 0.5]  Gain=1
  cfblk6 : DiscreteIntegrator  ICPrevOutput=DiscIntNeverNeededParam  ICPrevScaledInput=DiscIntNeverNeededParam
  cfblk7 : simulink/Discrete/Transfer Fcn Real Zero  ZeroZ=0.75  ICPrevInput=0.0  DoSatur=off
  cfblk8 : Reshape
  cfblk9 : Constant  Value=[-595215380.457802]  SampleTime=1
  cfblk2 : Outport
  wires:
  cfblk16/1 -> cfblk5/1
  cfblk6/1 -> cfblk8/1
  cfblk1/1 -> cfblk10/1(cfblk1)
  cfblk4/1 -> cfblk6/1
  cfblk8/1 -> cfblk3/1
  cfblk3/1 -> cfblk7/1
  cfblk5/1 -> cfblk2/1
  cfblk14/1 -> cfblk4/1
  cfblk10/1(cfblk2) -> cfblk11/1(cfblk1)
  cfblk15/1 -> cfblk11/2(cfblk8)
  cfblk9/1 -> cfblk11/3(cfblk9)

== system model/cfblk43 ==
  cfblk1 : Inport
  Action Port : ActionPort  ActionPortLabel=if(u1 >= 0)
  cfblk3 : Trigonometry
  cfblk4 : Gain  Gain=[-254919736.976658]
  cfblk5 : Subsystem
  cfblk6 : Subsystem
  cfblk8 : Delay
  cfblk9 : Delay
  cfblk2 : Outport
  cfblk7 : Outport  Port=2
  wires:
  cfblk4/1 -> cfblk6/1(cfblk1)
  cfblk1/1 -> cfblk7/1
  cfblk6/2(cfblk7) -> cfblk2/1
  cfblk3/1 -> cfblk5/2(cfblk11)
  cfblk5/2(cfblk12) -> cfblk4/1
  cfblk5/1(cfblk2) -> cfblk8/1
  cfblk8/1 -> cfblk3/1
  cfblk6/1(cfblk2) -> cfblk9/1
  cfblk9/1 -> cfblk5/1(cfblk1)

== system model/cfblk44 ==
  cfblk1 : Inport
  cfblk9 : Inport  Port=2
  Action Port : ActionPort  ActionPortLabel=else
  cfblk3 : Delay  ShowEnablePort=on
      settings: InputPortMap=u0,e6
  cfblk4 : DiscreteStateSpace  SampleTime=-1
  cfblk5 : UnaryMinus
  cfblk6 : Constant  Value=[-662447500.319375]  SampleTime=1
  cfblk7 : Constant  Value=[85355849.666719]  SampleTime=1
  cfblk8 : Subsystem
  cfblk2 : Outport
  wires:
  cfblk7/1 -> cfblk8/1(cfblk1)
  cfblk8/1(cfblk2) -> cfblk4/1
  cfblk1/1 -> cfblk3/1, cfblk8/4(cfblk14)
  cfblk4/1 -> cfblk5/1
  cfblk6/1 -> cfblk3/2
  cfblk9/1 -> cfblk8/2(cfblk12)
  cfblk3/1 -> cfblk8/3(cfblk13)
  cfblk5/1 -> cfblk2/1

== system model/cfblk33/cfblk5 ==
  cfblk1 : Inport
  cfblk8 : Inport  Port=2
  cfblk11 : Delay  SampleTime=1
  cfblk3 : PropagationDelay  SampleTime=1
  cfblk4 : simulink/Math Operations/MinMax Running Resettable  Function=min  vinit=0.0
  cfblk5 : simulink/Math Operations/MinMax Running Resettable  Function=min  vinit=0.0
  cfblk6 : PermuteDimensions
  cfblk7 : Constant  Value=[815652369.202711]  SampleTime=1
  cfblk2 : Outport
  cfblk9 : Outport  Port=2
  cfblk10 : Outport  Port=3
  wires:
  cfblk1/1 -> cfblk6/1, cfblk5/2
  cfblk7/1 -> cfblk9/1
  cfblk8/1 -> cfblk3/1
  cfblk6/1 -> cfblk5/1, cfblk2/1
  cfblk5/1 -> cfblk10/1, cfblk4/2
  cfblk4/1 -> cfblk3/2
  cfblk3/1 -> cfblk11/1
  cfblk11/1 -> cfblk4/1

== system model/cfblk33/cfblk6 ==
  cfblk1 : Inport
  cfblk3 : Sum  Inputs=+
  cfblk4 : Bias  Bias=[-522416102.489031]  SaturateOnIntegerOverflow=off
  cfblk5 : Sqrt  Operator=rSqrt  AlgorithmType=Newton-Raphson
  cfblk6 : Product
  cfblk7 : Constant  Value=[-798995891.397461]  SampleTime=1
  cfblk2 : Outport
  wires:
  cfblk7/1 -> cfblk4/1
  cfblk4/1 -> cfblk6/1
  cfblk3/1 -> cfblk6/2
  cfblk1/1 -> cfblk3/1
  cfblk5/1 -> cfblk2/1
  cfblk6/1 -> cfblk5/1

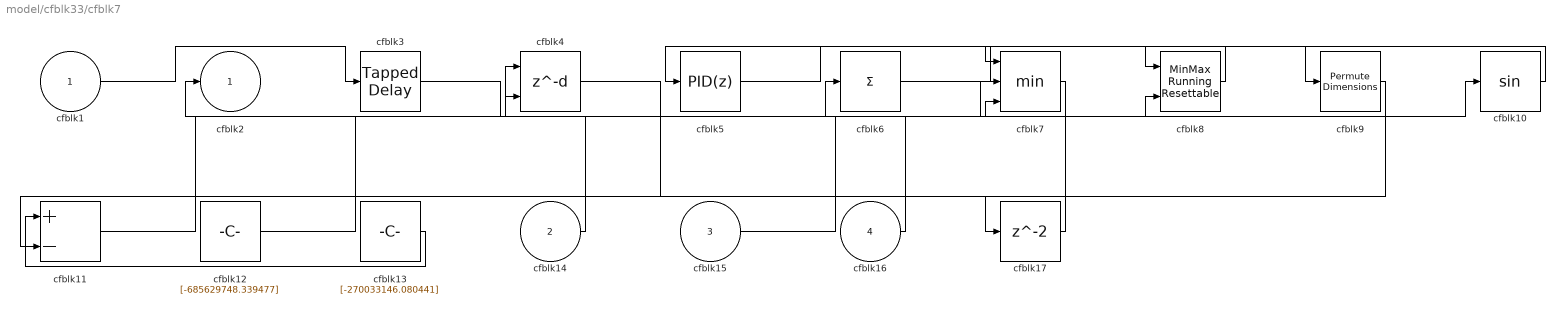
== system model/cfblk33/cfblk7 ==
  cfblk1 : Inport
  cfblk14 : Inport  Port=2
  cfblk15 : Inport  Port=3
  cfblk16 : Inport  Port=4
  cfblk10 : Trigonometry
  cfblk11 : Sum  Inputs=+-
  cfblk12 : Constant  Value=[-685629748.339477]  SampleTime=1
  cfblk13 : Constant  Value=[-270033146.080441]  SampleTime=1
  cfblk17 : Delay  SampleTime=1
  cfblk3 : simulink/Discrete/Tapped Delay  vinit=0.0  samptime=-1  NumDelays=1  DelayOrder=Oldest  includeCurrent=off
  cfblk4 : Delay  DelayLengthSource=Input port  SampleTime=1
      settings: InputPortMap=u0,p1
  cfblk5 : slpidlib/PID Controller  Controller=PID  Form=Parallel  TimeDomain=Discrete-time  UseExternalTs=off  SampleTime=1  IntegratorMethod=Forward Euler  FilterMethod=Forward Euler  ControllerParametersSource=internal  P=1  I=1  UseKiTs=off  D=0  N=100  UseFilter=on  TunerSelectOption=Transfer Function Based (PID Tuner App)  InitialConditionSource=internal  InitialConditionForIntegrator=0  InitialConditionForFilter=0  DifferentiatorICPrevScaledInput=0  ExternalReset=none  TrackingMode=off  Kt=1  LimitOutput=off  SatLimitsSource=internal  UpperSaturationLimit=inf  LowerSaturationLimit=-inf  LinearizeAsGain=off  AntiWindupMode=none  Kb=1  LimitIntegrator=off  UpperIntegratorSaturationLimit=inf  LowerIntegratorSaturationLimit=-inf  POutMin=[]  POutMax=[]  IOutMin=[]  IOutMax=[]  DOutMin=[]  DOutMax=[]  NOutMin=[]  NOutMax=[]  SumOutMin=[]  SumOutMax=[]  SaturationOutMin=[]  SaturationOutMax=[]  PParamMin=[]  PParamMax=[]  IParamMin=[]  IParamMax=[]  DParamMin=[]  DParamMax=[]  NParamMin=[]  NParamMax=[]  KbParamMin=[]  KbParamMax=[]  KtParamMin=[]  KtParamMax=[]  KbOutMin=[]  KbOutMax=[]  KtOutMin=[]  KtOutMax=[]  IntegratorOutMin=[]  IntegratorOutMax=[]  FilterOutMin=[]  FilterOutMax=[]  SumI1OutMin=[]  SumI1OutMax=[]  SumI2OutMin=[]  SumI2OutMax=[]  SumI3OutMin=[]  SumI3OutMax=[]  SumI4OutMin=[]  SumI4OutMax=[]  SumDOutMin=[]  SumDOutMax=[]  DifferentiatorOutMin=[]  DifferentiatorOutMax=[]  FilterDiffOutCoefMin=[]  FilterDiffOutCoefMax=[]  ReciprocalOutMin=[]  ReciprocalOutMax=[]  SumDenOutMin=[]  SumDenOutMax=[]  SumNumOutMin=[]  SumNumOutMax=[]  DivideOutMin=[]  DivideOutMax=[]  UdiffTsProdOutMin=[]  UdiffTsProdOutMax=[]  NTsProdOutMin=[]  NTsProdOutMax=[]  UintegralTsProdOutMin=[]  UintegralTsProdOutMax=[]  UngainTsProdOutMin=[]  UngainTsProdOutMax=[]  ClampingZeroOutDataTypeStr=Inherit: Inherit via back propagation  ClampingZeroOutMin=[]  ClampingZeroOutMax=[]  FilterDenConstantOutDataTypeStr=Inherit: Inherit via back propagation  FilterDenConstantOutMin=[]  FilterDenConstantOutMax=[]  PCopyOutDataTypeStr=Inherit: Inherit via back propagation  PCopyOutMin=[]  PCopyOutMax=[]  NCopyOutDataTypeStr=Inherit: Inherit via back propagation  NCopyOutMin=[]  NCopyOutMax=[]  IntegratorContinuousStateAttributes=''  IntegratorStateMustResolveToSignalObject=off  IntegratorRTWStateStorageClass=Auto  FilterContinuousStateAttributes=''  FilterStateMustResolveToSignalObject=off  FilterRTWStateStorageClass=Auto  ParallelPVariant=InternalParameters  IdealPVariant=Disabled  IVariant=InternalParameters  DVariant=InternalParameters  IntegratorVariant=Discrete  SatVariant=Disabled  AWVariant=Passthrough  PCopyVariant=Disabled  TRVariant=Disabled  FdbkBlocksVariant=Forward  IdealPFdbkVariant=Disabled  SatFdbkVariant=Disabled  DerivativeFilterVariant=ForwardEulerFilter  NVariant=InternalParameters  NCopyVariant=Disabled  FilterICVariant=InternalICsFilter  IntegratorICVariant=InternalICs  ExternalResetVariant=Disabled  TRSumVariant=Passthrough  SumFdbkVariant=Disabled  SumVariant=Sum_PID  TsampFilterVariant=InternalTs  TsampNgainVariant=Passthrough  TsampIntegralVariant=Disabled_SignalSpec  ExternalSaturationOutDataTypeStr=Inherit: Same as second input
      settings: LibrarySourceBlock=simulink/Discrete/Discrete PID Controller
  cfblk6 : Sum  Inputs=+
  cfblk7 : MinMax  Inputs=3
  cfblk8 : simulink/Math Operations/MinMax Running Resettable  Function=min  vinit=0.0
  cfblk9 : PermuteDimensions
  cfblk2 : Outport
  wires:
  cfblk11/1 -> cfblk10/1
  cfblk10/1 -> cfblk8/1
  cfblk14/1 -> cfblk2/1
  cfblk13/1 -> cfblk11/1
  cfblk9/1 -> cfblk11/2
  cfblk8/1 -> cfblk5/1
  cfblk15/1 -> cfblk8/2
  cfblk12/1 -> cfblk4/1
  cfblk16/1 -> cfblk6/1
  cfblk6/1 -> cfblk9/1
  cfblk1/1 -> cfblk3/1
  cfblk7/1 -> cfblk4/2
  cfblk5/1 -> cfblk7/1
  cfblk3/1 -> cfblk7/3
  cfblk4/1 -> cfblk17/1
  cfblk17/1 -> cfblk7/2

== system model/cfblk33/cfblk8 ==
  cfblk1 : Inport
  cfblk12 : Inport  Port=2
  cfblk13 : Inport  Port=3
  cfblk14 : Inport  Port=4
  cfblk10 : Constant  Value=[-544680512.953130]  SampleTime=1
  cfblk11 : Constant  Value=[506500576.835107]  SampleTime=1
  cfblk3 : UnitDelay  HasFrameUpgradeWarning=on
  cfblk4 : Delay  ShowEnablePort=on  SampleTime=1
      settings: InputPortMap=u0,e6
  cfblk5 : simulink/Discrete/Difference  ICPrevInput=0.0  OutMin=[]  OutMax=[]  OutDataTypeStr=Inherit: Inherit via back propagation  OutDataType=fixdt(1, 16)  OutScaling=2^-10  DoSatur=off
  cfblk6 : DiscreteTransferFcn  SampleTime=1
  cfblk7 : Signum
  cfblk8 : Sum  Inputs=|++
  cfblk9 : ComplexToRealImag
  cfblk2 : Outport
  cfblk15 : Outport  Port=2
  wires:
  cfblk4/1 -> cfblk7/1
  cfblk11/1 -> cfblk2/1
  cfblk8/1 -> cfblk15/1
  cfblk1/1 -> cfblk4/1
  cfblk3/1 -> cfblk6/1
  cfblk12/1 -> cfblk4/2
  cfblk14/1 -> cfblk3/1
  cfblk7/1 -> cfblk5/1
  cfblk13/1 -> cfblk8/1
  cfblk9/1 -> cfblk8/2
  cfblk6/1 -> cfblk9/1

== system model/cfblk34/cfblk12 ==
  cfblk1 : Inport
  cfblk9 : Inport  Port=2
  cfblk10 : Inport  Port=3
  cfblk11 : Inport  Port=4
  Action Port : ActionPort  ActionPortLabel=if(u1 >= 0)
  cfblk13 : Delay
  cfblk3 : Delay  DelayLengthSource=Input port
      settings: InputPortMap=u0,p1
  cfblk4 : DiscreteZeroPole  Poles=[0 0.5]  Gain=1  SampleTime=-1
  cfblk5 : Product  Inputs=*
  cfblk6 : Rounding
  cfblk7 : Constant  Value=[-74655399.879822]  SampleTime=1
  cfblk8 : Constant  Value=[-101411849.006172]  SampleTime=1
  cfblk2 : Outport
  cfblk12 : Outport  Port=2
  wires:
  cfblk6/1 -> cfblk5/1
  cfblk5/1 -> cfblk3/1
  cfblk3/1 -> cfblk4/1
  cfblk1/1 -> cfblk12/1
  cfblk7/1 -> cfblk6/1
  cfblk9/1 -> cfblk2/1
  cfblk4/1 -> cfblk13/1
  cfblk13/1 -> cfblk3/2

== system model/cfblk34/cfblk13 ==
  cfblk1 : Inport
  cfblk10 : Inport  Port=2
  cfblk11 : Inport  Port=3
  cfblk12 : Inport  Port=4
  cfblk13 : Inport  Port=5
  Action Port : ActionPort  ActionPortLabel=else
  cfblk3 : simulink/Discrete/Transfer Fcn Lead or Lag  PoleZ=0.95  ZeroZ=0.75  ICPrevOutput=0.0  ICPrevInput=0.0  DoSatur=off
  cfblk4 : slpidlib/PID Controller  Controller=PID  Form=Parallel  TimeDomain=Discrete-time  UseExternalTs=off  SampleTime=-1  IntegratorMethod=Forward Euler  FilterMethod=Forward Euler  ControllerParametersSource=internal  P=1  I=1  UseKiTs=off  D=0  N=100  UseFilter=on  TunerSelectOption=Transfer Function Based (PID Tuner App)  InitialConditionSource=internal  InitialConditionForIntegrator=0  InitialConditionForFilter=0  DifferentiatorICPrevScaledInput=0  ExternalReset=none  TrackingMode=off  Kt=1  LimitOutput=off  SatLimitsSource=internal  UpperSaturationLimit=inf  LowerSaturationLimit=-inf  LinearizeAsGain=off  AntiWindupMode=none  Kb=1  LimitIntegrator=off  UpperIntegratorSaturationLimit=inf  LowerIntegratorSaturationLimit=-inf  POutMin=[]  POutMax=[]  IOutMin=[]  IOutMax=[]  DOutMin=[]  DOutMax=[]  NOutMin=[]  NOutMax=[]  SumOutMin=[]  SumOutMax=[]  SaturationOutMin=[]  SaturationOutMax=[]  PParamMin=[]  PParamMax=[]  IParamMin=[]  IParamMax=[]  DParamMin=[]  DParamMax=[]  NParamMin=[]  NParamMax=[]  KbParamMin=[]  KbParamMax=[]  KtParamMin=[]  KtParamMax=[]  KbOutMin=[]  KbOutMax=[]  KtOutMin=[]  KtOutMax=[]  IntegratorOutMin=[]  IntegratorOutMax=[]  FilterOutMin=[]  FilterOutMax=[]  SumI1OutMin=[]  SumI1OutMax=[]  SumI2OutMin=[]  SumI2OutMax=[]  SumI3OutMin=[]  SumI3OutMax=[]  SumI4OutMin=[]  SumI4OutMax=[]  SumDOutMin=[]  SumDOutMax=[]  DifferentiatorOutMin=[]  DifferentiatorOutMax=[]  FilterDiffOutCoefMin=[]  FilterDiffOutCoefMax=[]  ReciprocalOutMin=[]  ReciprocalOutMax=[]  SumDenOutMin=[]  SumDenOutMax=[]  SumNumOutMin=[]  SumNumOutMax=[]  DivideOutMin=[]  DivideOutMax=[]  UdiffTsProdOutMin=[]  UdiffTsProdOutMax=[]  NTsProdOutMin=[]  NTsProdOutMax=[]  UintegralTsProdOutMin=[]  UintegralTsProdOutMax=[]  UngainTsProdOutMin=[]  UngainTsProdOutMax=[]  ClampingZeroOutDataTypeStr=Inherit: Inherit via back propagation  ClampingZeroOutMin=[]  ClampingZeroOutMax=[]  FilterDenConstantOutDataTypeStr=Inherit: Inherit via back propagation  FilterDenConstantOutMin=[]  FilterDenConstantOutMax=[]  PCopyOutDataTypeStr=Inherit: Inherit via back propagation  PCopyOutMin=[]  PCopyOutMax=[]  NCopyOutDataTypeStr=Inherit: Inherit via back propagation  NCopyOutMin=[]  NCopyOutMax=[]  IntegratorContinuousStateAttributes=''  IntegratorStateMustResolveToSignalObject=off  IntegratorRTWStateStorageClass=Auto  FilterContinuousStateAttributes=''  FilterStateMustResolveToSignalObject=off  FilterRTWStateStorageClass=Auto  ParallelPVariant=InternalParameters  IdealPVariant=Disabled  IVariant=InternalParameters  DVariant=InternalParameters  IntegratorVariant=Discrete  SatVariant=Disabled  AWVariant=Passthrough  PCopyVariant=Disabled  TRVariant=Disabled  FdbkBlocksVariant=Forward  IdealPFdbkVariant=Disabled  SatFdbkVariant=Disabled  DerivativeFilterVariant=ForwardEulerFilter  NVariant=InternalParameters  NCopyVariant=Disabled  FilterICVariant=InternalICsFilter  IntegratorICVariant=InternalICs  ExternalResetVariant=Disabled  TRSumVariant=Passthrough  SumFdbkVariant=Disabled  SumVariant=Sum_PID  TsampFilterVariant=InternalTs  TsampNgainVariant=Passthrough  TsampIntegralVariant=Disabled_SignalSpec  ExternalSaturationOutDataTypeStr=Inherit: Same as second input
      settings: LibrarySourceBlock=simulink/Discrete/Discrete PID Controller
  cfblk5 : Delay  ShowEnablePort=on
      settings: InputPortMap=u0,e6
  cfblk6 : Sum  Inputs=+-
  cfblk7 : UnaryMinus
  cfblk8 : Product
  cfblk9 : Constant  Value=[791996309.879964]  SampleTime=1
  cfblk2 : Outport
  cfblk14 : Outport  Port=2
  cfblk15 : Outport  Port=3
  wires:
  cfblk12/1 -> cfblk8/1
  cfblk9/1 -> cfblk4/1
  cfblk7/1 -> cfblk14/1
  cfblk8/1 -> cfblk2/1
  cfblk11/1 -> cfblk7/1
  cfblk4/1 -> cfblk3/1
  cfblk6/1 -> cfblk8/2
  cfblk3/1 -> cfblk5/1
  cfblk13/1 -> cfblk6/1
  cfblk1/1 -> cfblk15/1
  cfblk10/1 -> cfblk5/2
  cfblk5/1 -> cfblk6/2

== system model/cfblk34/cfblk7 ==
  cfblk1 : Inport
  cfblk7 : Inport  Port=2
  cfblk11 : Delay  SampleTime=1
  cfblk3 : DiscreteTransferFcn  SampleTime=1
  cfblk4 : DiscreteTransferFcn  SampleTime=1
  cfblk5 : slpidlib/PID Controller  Controller=PID  Form=Parallel  TimeDomain=Discrete-time  UseExternalTs=off  SampleTime=1  IntegratorMethod=Forward Euler  FilterMethod=Forward Euler  ControllerParametersSource=internal  P=1  I=1  UseKiTs=off  D=0  N=100  UseFilter=on  TunerSelectOption=Transfer Function Based (PID Tuner App)  InitialConditionSource=internal  InitialConditionForIntegrator=0  InitialConditionForFilter=0  DifferentiatorICPrevScaledInput=0  ExternalReset=none  TrackingMode=off  Kt=1  LimitOutput=off  SatLimitsSource=internal  UpperSaturationLimit=inf  LowerSaturationLimit=-inf  LinearizeAsGain=off  AntiWindupMode=none  Kb=1  LimitIntegrator=off  UpperIntegratorSaturationLimit=inf  LowerIntegratorSaturationLimit=-inf  POutMin=[]  POutMax=[]  IOutMin=[]  IOutMax=[]  DOutMin=[]  DOutMax=[]  NOutMin=[]  NOutMax=[]  SumOutMin=[]  SumOutMax=[]  SaturationOutMin=[]  SaturationOutMax=[]  PParamMin=[]  PParamMax=[]  IParamMin=[]  IParamMax=[]  DParamMin=[]  DParamMax=[]  NParamMin=[]  NParamMax=[]  KbParamMin=[]  KbParamMax=[]  KtParamMin=[]  KtParamMax=[]  KbOutMin=[]  KbOutMax=[]  KtOutMin=[]  KtOutMax=[]  IntegratorOutMin=[]  IntegratorOutMax=[]  FilterOutMin=[]  FilterOutMax=[]  SumI1OutMin=[]  SumI1OutMax=[]  SumI2OutMin=[]  SumI2OutMax=[]  SumI3OutMin=[]  SumI3OutMax=[]  SumI4OutMin=[]  SumI4OutMax=[]  SumDOutMin=[]  SumDOutMax=[]  DifferentiatorOutMin=[]  DifferentiatorOutMax=[]  FilterDiffOutCoefMin=[]  FilterDiffOutCoefMax=[]  ReciprocalOutMin=[]  ReciprocalOutMax=[]  SumDenOutMin=[]  SumDenOutMax=[]  SumNumOutMin=[]  SumNumOutMax=[]  DivideOutMin=[]  DivideOutMax=[]  UdiffTsProdOutMin=[]  UdiffTsProdOutMax=[]  NTsProdOutMin=[]  NTsProdOutMax=[]  UintegralTsProdOutMin=[]  UintegralTsProdOutMax=[]  UngainTsProdOutMin=[]  UngainTsProdOutMax=[]  ClampingZeroOutDataTypeStr=Inherit: Inherit via back propagation  ClampingZeroOutMin=[]  ClampingZeroOutMax=[]  FilterDenConstantOutDataTypeStr=Inherit: Inherit via back propagation  FilterDenConstantOutMin=[]  FilterDenConstantOutMax=[]  PCopyOutDataTypeStr=Inherit: Inherit via back propagation  PCopyOutMin=[]  PCopyOutMax=[]  NCopyOutDataTypeStr=Inherit: Inherit via back propagation  NCopyOutMin=[]  NCopyOutMax=[]  IntegratorContinuousStateAttributes=''  IntegratorStateMustResolveToSignalObject=off  IntegratorRTWStateStorageClass=Auto  FilterContinuousStateAttributes=''  FilterStateMustResolveToSignalObject=off  FilterRTWStateStorageClass=Auto  ParallelPVariant=InternalParameters  IdealPVariant=Disabled  IVariant=InternalParameters  DVariant=InternalParameters  IntegratorVariant=Discrete  SatVariant=Disabled  AWVariant=Passthrough  PCopyVariant=Disabled  TRVariant=Disabled  FdbkBlocksVariant=Forward  IdealPFdbkVariant=Disabled  SatFdbkVariant=Disabled  DerivativeFilterVariant=ForwardEulerFilter  NVariant=InternalParameters  NCopyVariant=Disabled  FilterICVariant=InternalICsFilter  IntegratorICVariant=InternalICs  ExternalResetVariant=Disabled  TRSumVariant=Passthrough  SumFdbkVariant=Disabled  SumVariant=Sum_PID  TsampFilterVariant=InternalTs  TsampNgainVariant=Passthrough  TsampIntegralVariant=Disabled_SignalSpec  ExternalSaturationOutDataTypeStr=Inherit: Same as second input
      settings: LibrarySourceBlock=simulink/Discrete/Discrete PID Controller
  cfblk6 : Sqrt
  cfblk2 : Outport
  cfblk8 : Outport  Port=2
  cfblk9 : Outport  Port=3
  cfblk10 : Outport  Port=4
  wires:
  cfblk3/1 -> cfblk10/1, cfblk5/1
  cfblk6/1 -> cfblk9/1, cfblk2/1
  cfblk5/1 -> cfblk4/1
  cfblk1/1 -> cfblk6/1
  cfblk7/1 -> cfblk8/1
  cfblk4/1 -> cfblk11/1
  cfblk11/1 -> cfblk3/1

== system model/cfblk34/cfblk8 ==
  cfblk1 : Inport
  cfblk11 : Delay  SampleTime=1
  cfblk12 : Delay  SampleTime=1
  cfblk3 : Delay  DelayLengthSource=Input port  SampleTime=1
      settings: InputPortMap=u0,p1
  cfblk4 : simulink/Discrete/Transfer Fcn First Order  PoleZ=0.95  ICPrevOutput=0.0  DoSatur=off
  cfblk5 : Reshape
  cfblk6 : Rounding
  cfblk7 : Product  Inputs=*
  cfblk8 : DotProduct  OutDataTypeStr=Inherit: Inherit via internal rule
  cfblk2 : Outport
  cfblk9 : Outport  Port=2
  cfblk10 : Outport  Port=3
  wires:
  cfblk3/1 -> cfblk7/1, cfblk6/1
  cfblk8/1 -> cfblk4/1
  cfblk1/1 -> cfblk3/1
  cfblk7/1 -> cfblk5/1, cfblk2/1, cfblk8/2
  cfblk5/1 -> cfblk10/1
  cfblk6/1 -> cfblk9/1, cfblk12/1
  cfblk4/1 -> cfblk11/1
  cfblk11/1 -> cfblk8/1
  cfblk12/1 -> cfblk3/2

== system model/cfblk34/cfblk9 ==
  cfblk1 : Inport
  cfblk6 : Inport  Port=2
  cfblk7 : Inport  Port=3
  cfblk10 : Delay  SampleTime=1
  cfblk3 : Rounding
  cfblk4 : Reshape
  cfblk5 : Sum  Inputs=+
  cfblk2 : Outport
  cfblk8 : Outport  Port=2
  cfblk9 : Outport  Port=3
  wires:
  cfblk1/1 -> cfblk3/1
  cfblk4/1 -> cfblk5/1
  cfblk3/1 -> cfblk9/1
  cfblk6/1 -> cfblk2/1
  cfblk7/1 -> cfblk8/1
  cfblk5/1 -> cfblk10/1
  cfblk10/1 -> cfblk4/1

== system model/cfblk35/cfblk10 ==
  cfblk1 : Inport
  cfblk10 : Inport  Port=2
  cfblk11 : Inport  Port=3
  cfblk12 : Inport  Port=4
  cfblk13 : Inport  Port=5
  cfblk14 : Inport  Port=6
  cfblk15 : Inport  Port=7
  cfblk3 : PropagationDelay  SampleTime=1
  cfblk4 : Sqrt
  cfblk5 : Product  Inputs=**
  cfblk6 : Signum
  cfblk7 : Sqrt  Operator=rSqrt  AlgorithmType=Newton-Raphson
  cfblk8 : Constant  Value=[604776771.456297]  SampleTime=1
  cfblk9 : Constant  Value=[-246743620.445108]  SampleTime=1
  cfblk2 : Outport
  wires:
  cfblk15/1 -> cfblk6/1
  cfblk11/1 -> cfblk4/1
  cfblk5/1 -> cfblk7/1
  cfblk10/1 -> cfblk3/1
  cfblk1/1 -> cfblk5/1
  cfblk6/1 -> cfblk5/2
  cfblk8/1 -> cfblk3/2
  cfblk7/1 -> cfblk2/1
